simulink model "DF_Hinf_tuning"  (R2016b)
settings: Solver=VariableStepAuto  StartTime=0.0  StopTime=20  RelTol=1e-3  EnableMultiTasking=on
values from neighbouring files (symbols this model uses):
  Ap = Aa    [main.m]
  Bd = [eye(6);zeros(3,6)]    [main.m]
  Bp = Ba    [main.m]
  Cp = f_select_matrix([1 2 3 9],9)    [main.m]
  KF = Kblock.KF.d    [main.m]
  KI = Kblock.KI.d    [main.m]
undefined symbols (not defined in the file): Cs, Ds
libraries: simulink x6
settings Model: Creator=wangxiaoliang  LastModifiedBy=user
settings OptimizationCC: LifeSpan=inf
settings DebuggingCC: SFUnexpectedBacktrackingDiag=warning  SFNoUnconditionalDefaultTransitionDiag=warning  SFExecutionAtInitializationDiag=none
settings GRTTargetCC: TargetLangStandard=C89/C90 (ANSI)  GeneratePreprocessorConditionals=Disable all
settings ConfigComp: CovMetricSettings=dw  CovHtmlReporting=on  CovSaveCumulativeToWorkspaceVar=on  CovSaveSingleToWorkspaceVar=on  CovExternalEMLEnable=off

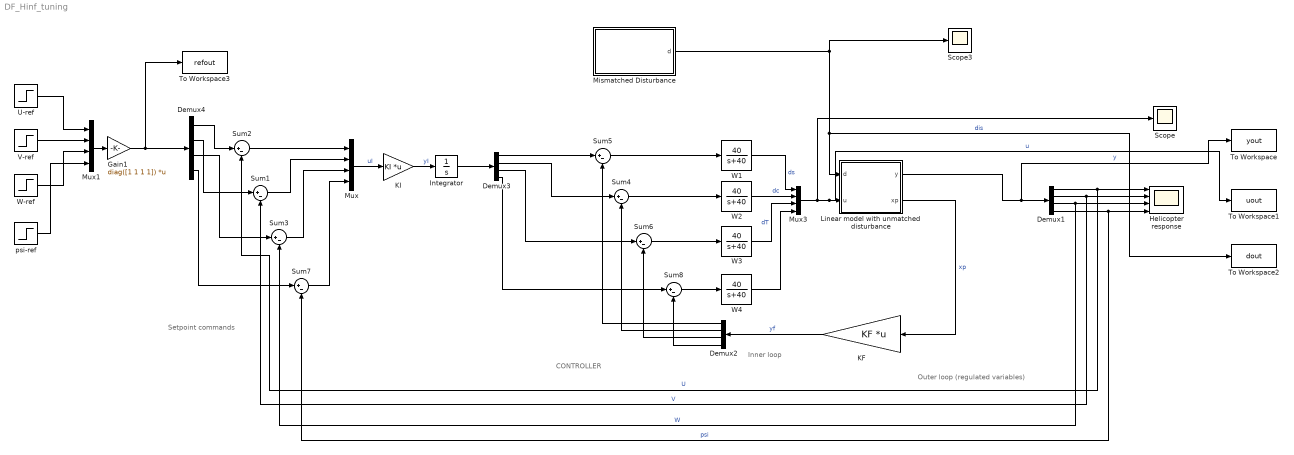
== system DF_Hinf_tuning ==
  note: CONTROLLER
  note: Setpoint
      | commands
  note: Inner loop
  note: Outer loop (regulated variables)
  Demux{1..4} (4 alike) : Demux
  Gain1 : Gain  Gain=diag([1 1 1 1])  Multiplication=Matrix(K*u)
  Helicopter response : Scope  NumInputPorts=4
  Integrator : Integrator
  KF : Gain  Gain=KF  Multiplication=Matrix(K*u) (u vector)
  KI : Gain  Gain=KI  Multiplication=Matrix(K*u)
  Linear model with unmatched disturbance : Subsystem  mask{Ap=Ap, Bp=Bp, Bd=Bd, Cp=Cp, Cs=Cs, Ds=Ds}
  Mismatched Disturbance : Subsystem  mask{wb=2.5, k=0.4, Ts=0.001}
      mask prompts: wb "wb (Filter bandwidth)"; k "k (Signal standard deviation)"; Ts "Ts (Sample time)"
  Mux : Mux
  Mux1 : Mux
  Mux3 : Mux
  Scope : Scope
  Scope3 : Scope
  Sum{1..8} (8 alike) : Sum  Inputs=|+-
  To Workspace : ToWorkspace  VariableName=yout  SaveFormat=Timeseries  SampleTime=-1
  To Workspace1 : ToWorkspace  VariableName=uout  SaveFormat=Timeseries  SampleTime=-1
  To Workspace2 : ToWorkspace  VariableName=dout  SaveFormat=Timeseries  SampleTime=-1
  To Workspace3 : ToWorkspace  VariableName=refout  SaveFormat=Timeseries  SampleTime=-1
  U-ref : Step  Time=0  SampleTime=0
  V-ref : Step  Time=0  SampleTime=0
  W-ref : Step  Time=0  SampleTime=0
  W{1..4} (4 alike) : TransferFcn  Numerator=[40]  Denominator=[1 40]
  psi-ref : Step  Time=0  SampleTime=0
  wires:
  Mux3/1 -> Scope/1, To Workspace1/1, Linear model with unmatched disturbance/2(u)  "u"
  W3/1 -> Mux3/3  "dT"
  W2/1 -> Mux3/2  "dc"
  W1/1 -> Mux3/1  "ds"
  Linear model with unmatched disturbance/2(xp) -> KF/1  "xp"
  Demux1/1 -> Sum2/2, Helicopter response/1  "U"
  Demux1/2 -> Sum1/2, Helicopter response/2  "V"
  Demux1/3 -> Sum3/2, Helicopter response/3  "W"
  Sum2/1 -> Mux/1
  KF/1 -> Demux2/1  "yf"
  Sum1/1 -> Mux/2
  Sum3/1 -> Mux/3
  Demux2/1 -> Sum5/2
  Demux2/2 -> Sum4/2
  Demux2/3 -> Sum6/2
  Linear model with unmatched disturbance/1(y) -> To Workspace/1, Demux1/1  "y"
  Sum5/1 -> W1/1
  Sum4/1 -> W2/1
  Sum6/1 -> W3/1
  Sum7/1 -> Mux/4
  Demux2/4 -> Sum8/2
  Sum8/1 -> W4/1
  W4/1 -> Mux3/4
  Demux1/4 -> Sum7/2, Helicopter response/4  "psi"
  Mux/1 -> KI/1  "uI"
  KI/1 -> Integrator/1  "yI"
  Integrator/1 -> Demux3/1
  Demux3/1 -> Sum5/1
  Demux3/2 -> Sum4/1
  Demux3/3 -> Sum6/1
  Demux3/4 -> Sum8/1
  U-ref/1 -> Mux1/1
  V-ref/1 -> Mux1/2
  W-ref/1 -> Mux1/3
  psi-ref/1 -> Mux1/4
  Mux1/1 -> Gain1/1
  Demux4/1 -> Sum2/1
  Demux4/2 -> Sum1/1
  Demux4/3 -> Sum3/1
  Demux4/4 -> Sum7/1
  Gain1/1 -> Demux4/1, To Workspace3/1
  Mismatched Disturbance/1(d) -> Scope3/1, To Workspace2/1, Linear model with unmatched disturbance/1(d)  "dis"

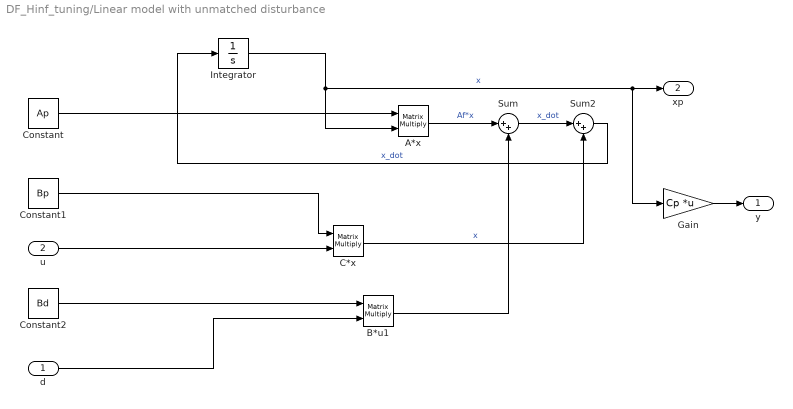
== system DF_Hinf_tuning/Linear model with unmatched disturbance ==
  d : Inport
  u : Inport  Port=2
  A*x : Product  Multiplication=Matrix(*)
  B*u1 : Product  Multiplication=Matrix(*)
  C*x : Product  Multiplication=Matrix(*)
  Constant : Constant  Value=Ap
  Constant1 : Constant  Value=Bp
  Constant2 : Constant  Value=Bd
  Gain : Gain  Gain=Cp  Multiplication=Matrix(K*u)
  Integrator : Integrator  UpperSaturationLimit=1000  LowerSaturationLimit=-1000
  Sum : Sum  Inputs=|++
  Sum2 : Sum  Inputs=|++
  y : Outport
  xp : Outport  Port=2
  wires:
  A*x/1 -> Sum/1  "Af*x"
  C*x/1 -> Sum2/2  "x"
  Integrator/1 -> xp/1, Gain/1, A*x/2  "x"
  Sum2/1 -> Integrator/1  "x_dot"
  Constant/1 -> A*x/1
  Constant2/1 -> B*u1/1
  B*u1/1 -> Sum/2
  Sum/1 -> Sum2/1  "x_dot"
  Constant1/1 -> C*x/1
  Gain/1 -> y/1
  u/1 -> C*x/2
  d/1 -> B*u1/2

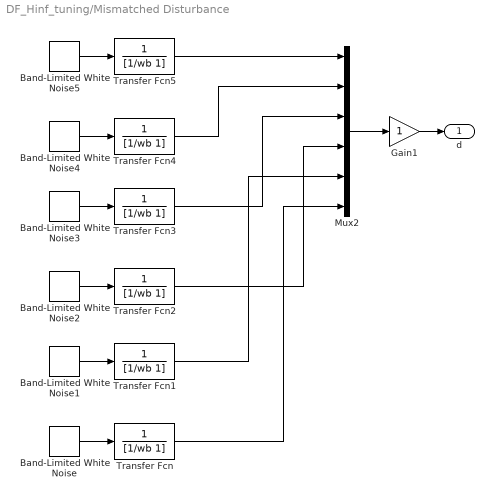
== system DF_Hinf_tuning/Mismatched Disturbance ==
  Band-Limited White Noise : simulink/Sources/Band-Limited White Noise  Cov=2*k^2/wb  Ts=Ts  seed=[23345]
  Band-Limited White Noise1 : simulink/Sources/Band-Limited White Noise  Cov=2*k^2/wb  Ts=Ts  seed=[23344]
  Band-Limited White Noise2 : simulink/Sources/Band-Limited White Noise  Cov=2*k^2/wb  Ts=Ts  seed=[23341]
  Band-Limited White Noise3 : simulink/Sources/Band-Limited White Noise  Cov=2*k^2/wb  Ts=Ts  seed=[23340]
  Band-Limited White Noise4 : simulink/Sources/Band-Limited White Noise  Cov=2*k^2/wb  Ts=Ts  seed=[23343]
  Band-Limited White Noise5 : simulink/Sources/Band-Limited White Noise  Cov=2*k^2/wb  Ts=Ts  seed=[23342]
  Gain1 : Gain
  Mux2 : Mux  Inputs=6
  Transfer Fcn{,1..5} (6 alike) : TransferFcn  Denominator=[1/wb 1]
  d : Outport
  wires:
  Transfer Fcn3/1 -> Mux2/3
  Mux2/1 -> Gain1/1
  Band-Limited White Noise3/1 -> Transfer Fcn3/1
  Band-Limited White Noise2/1 -> Transfer Fcn2/1
  Band-Limited White Noise1/1 -> Transfer Fcn1/1
  Transfer Fcn4/1 -> Mux2/2
  Transfer Fcn1/1 -> Mux2/5
  Transfer Fcn5/1 -> Mux2/1
  Transfer Fcn2/1 -> Mux2/4
  Transfer Fcn/1 -> Mux2/6
  Band-Limited White Noise/1 -> Transfer Fcn/1
  Band-Limited White Noise4/1 -> Transfer Fcn4/1
  Band-Limited White Noise5/1 -> Transfer Fcn5/1
  Gain1/1 -> d/1
